simulink model "PARCIAL_2_Sotar_E4"  (R2018a)
settings: Solver=ode15s  StartTime=0.0  StopTime=20  RelTol=1e-3
values from neighbouring files (symbols this model uses):
  L = lqr(A', C', Q, R)'    [PARCIAL_2_E3_script_2p.m]    (also in PARCIAL_2_Sotar_E3.m)
libraries: fl_lib x14, nesl_utility x12, sdolib x5, simulink x5
settings Model: Creator=joses  LastModifiedBy=mluser

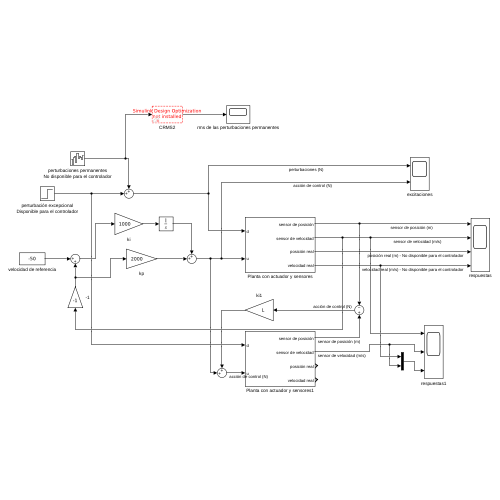
[thumbnail: Simulink's stored preview of the top-level diagram]
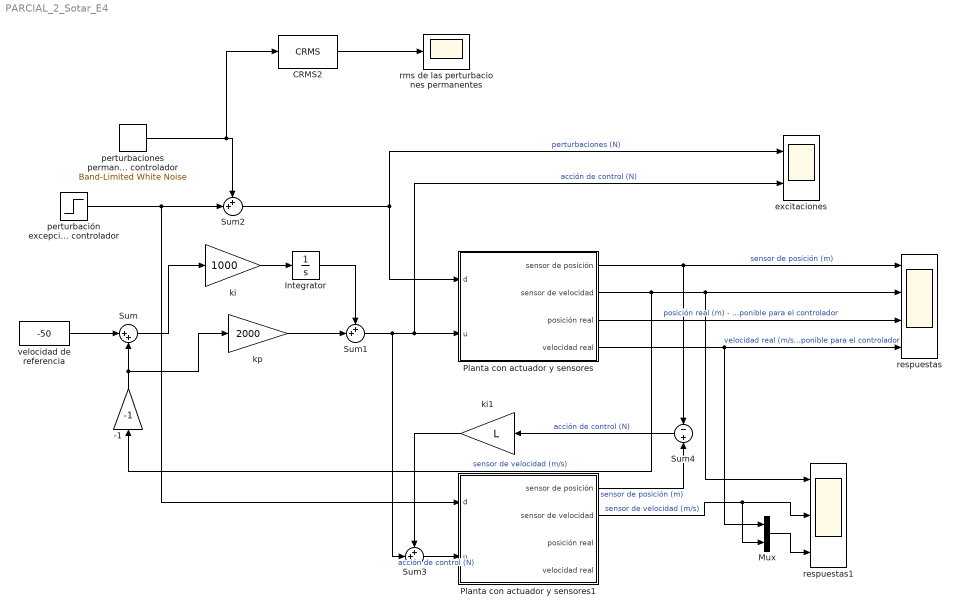
== system PARCIAL_2_Sotar_E4 ==
  -1 : Gain  Gain=-1
  CRMS2 : sdolib/RMS Blocks/CRMS
  Integrator : Integrator
  Mux : Mux  Inputs=2
  Planta con actuador y sensores : Subsystem
  Planta con actuador y sensores1 : Subsystem
  Sum : Sum  Inputs=|++
  Sum1 : Sum  Inputs=++|
  Sum2 : Sum  Inputs=++|
  Sum3 : Sum  Inputs=++|
  Sum4 : Sum  Inputs=-+
  excitaciones : Scope  NumInputPorts=2
  ki : Gain  Gain=1000
  ki1 : Gain  Gain=L
  kp : Gain  Gain=2000
  perturbaciones permanentes No disponible para el controlador : simulink/Sources/Band-Limited White Noise  Cov=100000  Ts=0.01  seed=[23341]
  perturbación excepcional Disponible para el controlador : Step  Time=10  After=20000  SampleTime=0
  respuestas : Scope  NumInputPorts=4
  respuestas1 : Scope  NumInputPorts=3
  rms de las perturbaciones permanentes : Scope
  velocidad de referencia : Constant  Value=-50
  wires:
  Planta con actuador y sensores/2(sensor de velocidad) -> -1/1, respuestas1/1, respuestas/2  "sensor de velocidad (m/s)"
  Planta con actuador y sensores/1(sensor de posición) -> Sum4/1, respuestas/1  "sensor de posición (m)"
  velocidad de referencia/1 -> Sum/1
  Sum/1 -> ki/1
  kp/1 -> Sum1/2
  Planta con actuador y sensores/3(posición real) -> respuestas/3  "posición real (m) - No disponible para el controlador"
  Planta con actuador y sensores/4(velocidad real) -> respuestas/4, Mux/1  "velocidad real (m/s) - No disponible para el controlador"
  Sum1/1 -> Sum3/2, excitaciones/2, Planta con actuador y sensores/2(u)  "acción de control (N)"
  Integrator/1 -> Sum1/1
  ki/1 -> Integrator/1
  perturbación excepcional Disponible para el controlador/1 -> Planta con actuador y sensores1/1(d), Sum2/2
  Sum2/1 -> excitaciones/1, Planta con actuador y sensores/1(d)  "perturbaciones (N)"
  -1/1 -> kp/1, Sum/2
  CRMS2/1 -> rms de las perturbaciones permanentes/1
  perturbaciones permanentes No disponible para el controlador/1 -> CRMS2/1, Sum2/1
  ki1/1 -> Sum3/1
  Planta con actuador y sensores1/1(sensor de posición) -> Sum4/2  "sensor de posición (m)"
  Sum4/1 -> ki1/1  "acción de control (N)"
  Sum3/1 -> Planta con actuador y sensores1/2(u)  "acción de control (N)"
  Planta con actuador y sensores1/2(sensor de velocidad) -> Mux/2, respuestas1/2  "sensor de velocidad (m/s)"
  Mux/1 -> respuestas1/3

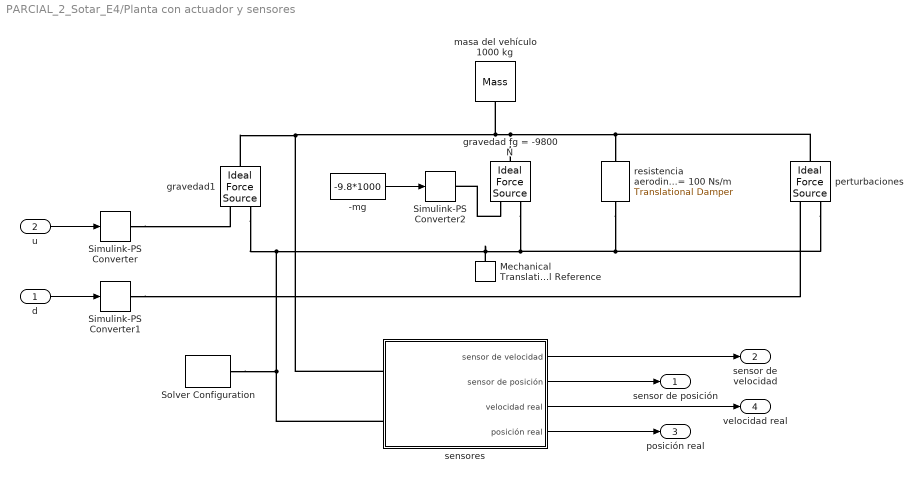
== system PARCIAL_2_Sotar_E4/Planta con actuador y sensores ==
  d : Inport
  u : Inport  Port=2
  -mg : Constant  Value=-9.8*1000
  Mechanical Translational Reference : fl_lib/Mechanical/Translational Elements/Mechanical Translational Reference
  Simulink-PS Converter : nesl_utility/Simulink-PS Converter  PhysicalDomain=network_engine_domain  SubClassName=ps_input  LeftPortType=input  RightPortType=output  PseudoPeriodic=off  Frequencies=[]  NoiseDistribution=none  NoiseParameters=[]  Unit=1  AffineConversion=off  FilteringAndDerivatives=provide  SimscapeFilterOrder=1  InputFilterTimeConstant=0.001  UdotUserProvided=0
  Simulink-PS Converter1 : nesl_utility/Simulink-PS Converter  PhysicalDomain=network_engine_domain  SubClassName=ps_input  LeftPortType=input  RightPortType=output  PseudoPeriodic=off  Frequencies=[]  NoiseDistribution=none  NoiseParameters=[]  Unit=1  AffineConversion=off  FilteringAndDerivatives=provide  SimscapeFilterOrder=1  InputFilterTimeConstant=0.001  UdotUserProvided=0
  Simulink-PS Converter2 : nesl_utility/Simulink-PS Converter  PhysicalDomain=network_engine_domain  SubClassName=ps_input  LeftPortType=input  RightPortType=output  PseudoPeriodic=off  Frequencies=[]  NoiseDistribution=none  NoiseParameters=[]  Unit=1  AffineConversion=off  FilteringAndDerivatives=provide  SimscapeFilterOrder=1  InputFilterTimeConstant=0.001  UdotUserProvided=0
  Solver Configuration : nesl_utility/Solver Configuration  PhysicalDomain=network_engine_domain  SubClassName=solver  LeftPortType=input  RightPortType=generic  Tones=[]  Harmonics=[]  SimulateNoise=off  Profile=off  UseLocalSampling=off  EnableSwitchedLinearOptims=on  FrequencyDomain=off  UseCCode=off  RelTol=0.001  AbsTol=1e-06  MinStep=1e-09  ToWorkspace=off  RevertToSquareIcSolve=off  NumHomotopyIterations=100  PhasorMode=off  PhasorModeNumHarmonics=1  DoDC=off  ResidualTolerance=1e-09  UseLocalSolver=off  LocalSolverChoice=NE_BACKWARD_EULER_ADVANCER  LocalSolverSampleTime=0.001  DoFixedCost=off  MaxNonlinIter=3  MaxModeIter=2  LinearAlgebra=Sparse  EquationFormulation=NE_TIME_EF  DelaysMemoryBudget=1024  AutomaticFiltering=on  FilteringTimeConstant=0.001
  gravedad fg = -9800 N : fl_lib/Mechanical/Mechanical Sources/Ideal Force Source
  gravedad1 : fl_lib/Mechanical/Mechanical Sources/Ideal Force Source
  masa del vehículo 1000 kg : fl_lib/Mechanical/Translational Elements/Mass  mass=1000 kg  v_specify=off  v_priority=High  v=0 m/s  v_nominal_specify=off  v_nominal_unit=m/s  v_nominal_value=1  f_specify=off  f_priority=None  f=0 N  f_nominal_specify=off  f_nominal_unit=N  f_nominal_value=1
  perturbaciones : fl_lib/Mechanical/Mechanical Sources/Ideal Force Source
  resistencia aerodinámica c = 100 Ns/m : fl_lib/Mechanical/Translational Elements/Translational Damper  D=100 N/(m/s)  v_specify=off  v_priority=None  v=0 m/s  v_nominal_specify=off  v_nominal_unit=m/s  v_nominal_value=1  f_specify=off  f_priority=None  f=0 N  f_nominal_specify=off  f_nominal_unit=N  f_nominal_value=1
  sensores : Subsystem
  sensor de posición : Outport  VectorParamsAs1DForOutWhenUnconnected=off
  sensor de velocidad : Outport  Port=2  VectorParamsAs1DForOutWhenUnconnected=off
  posición real : Outport  Port=3  VectorParamsAs1DForOutWhenUnconnected=off
  velocidad real : Outport  Port=4  VectorParamsAs1DForOutWhenUnconnected=off
  wires:
  sensores/2(sensor de posición) -> sensor de posición/1
  sensores/1(sensor de velocidad) -> sensor de velocidad/1
  d/1 -> Simulink-PS Converter1/1
  u/1 -> Simulink-PS Converter/1
  -mg/1 -> Simulink-PS Converter2/1
  sensores/3(velocidad real) -> velocidad real/1
  sensores/4(posición real) -> posición real/1
  connections:
  masa del vehículo 1000 kg/LConn1 -- gravedad1/LConn1 -- sensores/LConn1 -- gravedad fg = -9800 N/LConn1 -- perturbaciones/LConn1 -- resistencia aerodinámica c = 100 Ns/m/RConn1
  Simulink-PS Converter1/RConn1 -- perturbaciones/RConn1
  Mechanical Translational Reference/LConn1 -- gravedad1/RConn2 -- Solver Configuration/RConn1 -- sensores/LConn2 -- resistencia aerodinámica c = 100 Ns/m/LConn1 -- perturbaciones/RConn2 -- gravedad fg = -9800 N/RConn2
  Simulink-PS Converter/RConn1 -- gravedad1/RConn1
  gravedad fg = -9800 N/RConn1 -- Simulink-PS Converter2/RConn1

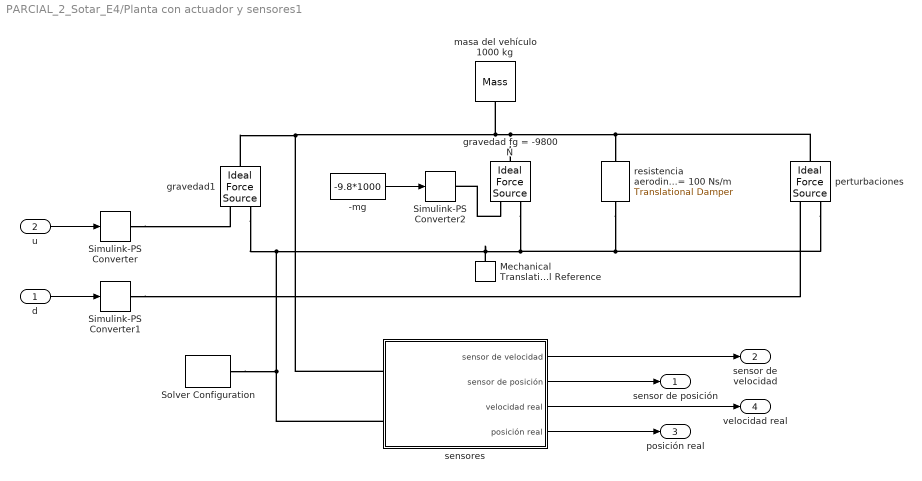
== system PARCIAL_2_Sotar_E4/Planta con actuador y sensores1 ==
  d : Inport
  u : Inport  Port=2
  -mg : Constant  Value=-9.8*1000
  Mechanical Translational Reference : fl_lib/Mechanical/Translational Elements/Mechanical Translational Reference
  Simulink-PS Converter : nesl_utility/Simulink-PS Converter  PhysicalDomain=network_engine_domain  SubClassName=ps_input  LeftPortType=input  RightPortType=output  PseudoPeriodic=off  Frequencies=[]  NoiseDistribution=none  NoiseParameters=[]  Unit=1  AffineConversion=off  FilteringAndDerivatives=provide  SimscapeFilterOrder=1  InputFilterTimeConstant=0.001  UdotUserProvided=0
  Simulink-PS Converter1 : nesl_utility/Simulink-PS Converter  PhysicalDomain=network_engine_domain  SubClassName=ps_input  LeftPortType=input  RightPortType=output  PseudoPeriodic=off  Frequencies=[]  NoiseDistribution=none  NoiseParameters=[]  Unit=1  AffineConversion=off  FilteringAndDerivatives=provide  SimscapeFilterOrder=1  InputFilterTimeConstant=0.001  UdotUserProvided=0
  Simulink-PS Converter2 : nesl_utility/Simulink-PS Converter  PhysicalDomain=network_engine_domain  SubClassName=ps_input  LeftPortType=input  RightPortType=output  PseudoPeriodic=off  Frequencies=[]  NoiseDistribution=none  NoiseParameters=[]  Unit=1  AffineConversion=off  FilteringAndDerivatives=provide  SimscapeFilterOrder=1  InputFilterTimeConstant=0.001  UdotUserProvided=0
  Solver Configuration : nesl_utility/Solver Configuration  PhysicalDomain=network_engine_domain  SubClassName=solver  LeftPortType=input  RightPortType=generic  Tones=[]  Harmonics=[]  SimulateNoise=off  Profile=off  UseLocalSampling=off  EnableSwitchedLinearOptims=on  FrequencyDomain=off  UseCCode=off  RelTol=0.001  AbsTol=1e-06  MinStep=1e-09  ToWorkspace=off  RevertToSquareIcSolve=off  NumHomotopyIterations=100  PhasorMode=off  PhasorModeNumHarmonics=1  DoDC=off  ResidualTolerance=1e-09  UseLocalSolver=off  LocalSolverChoice=NE_BACKWARD_EULER_ADVANCER  LocalSolverSampleTime=0.001  DoFixedCost=off  MaxNonlinIter=3  MaxModeIter=2  LinearAlgebra=Sparse  EquationFormulation=NE_TIME_EF  DelaysMemoryBudget=1024  AutomaticFiltering=on  FilteringTimeConstant=0.001
  gravedad fg = -9800 N : fl_lib/Mechanical/Mechanical Sources/Ideal Force Source
  gravedad1 : fl_lib/Mechanical/Mechanical Sources/Ideal Force Source
  masa del vehículo 1000 kg : fl_lib/Mechanical/Translational Elements/Mass  mass=1000 kg  v_specify=off  v_priority=High  v=0 m/s  v_nominal_specify=off  v_nominal_unit=m/s  v_nominal_value=1  f_specify=off  f_priority=None  f=0 N  f_nominal_specify=off  f_nominal_unit=N  f_nominal_value=1
  perturbaciones : fl_lib/Mechanical/Mechanical Sources/Ideal Force Source
  resistencia aerodinámica c = 100 Ns/m : fl_lib/Mechanical/Translational Elements/Translational Damper  D=100 N/(m/s)  v_specify=off  v_priority=None  v=0 m/s  v_nominal_specify=off  v_nominal_unit=m/s  v_nominal_value=1  f_specify=off  f_priority=None  f=0 N  f_nominal_specify=off  f_nominal_unit=N  f_nominal_value=1
  sensores : Subsystem
  sensor de posición : Outport  VectorParamsAs1DForOutWhenUnconnected=off
  sensor de velocidad : Outport  Port=2  VectorParamsAs1DForOutWhenUnconnected=off
  posición real : Outport  Port=3  VectorParamsAs1DForOutWhenUnconnected=off
  velocidad real : Outport  Port=4  VectorParamsAs1DForOutWhenUnconnected=off
  wires:
  sensores/2(sensor de posición) -> sensor de posición/1
  sensores/1(sensor de velocidad) -> sensor de velocidad/1
  d/1 -> Simulink-PS Converter1/1
  u/1 -> Simulink-PS Converter/1
  -mg/1 -> Simulink-PS Converter2/1
  sensores/3(velocidad real) -> velocidad real/1
  sensores/4(posición real) -> posición real/1
  connections:
  masa del vehículo 1000 kg/LConn1 -- gravedad1/LConn1 -- sensores/LConn1 -- gravedad fg = -9800 N/LConn1 -- perturbaciones/LConn1 -- resistencia aerodinámica c = 100 Ns/m/RConn1
  Simulink-PS Converter1/RConn1 -- perturbaciones/RConn1
  Mechanical Translational Reference/LConn1 -- gravedad1/RConn2 -- Solver Configuration/RConn1 -- sensores/LConn2 -- resistencia aerodinámica c = 100 Ns/m/LConn1 -- perturbaciones/RConn2 -- gravedad fg = -9800 N/RConn2
  Simulink-PS Converter/RConn1 -- gravedad1/RConn1
  gravedad fg = -9800 N/RConn1 -- Simulink-PS Converter2/RConn1

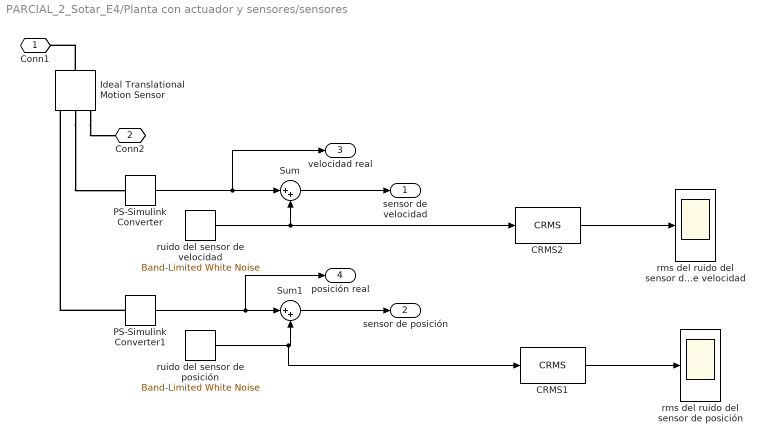
== system PARCIAL_2_Sotar_E4/Planta con actuador y sensores/sensores ==
  CRMS1 : sdolib/RMS Blocks/CRMS
  CRMS2 : sdolib/RMS Blocks/CRMS
  Ideal Translational Motion Sensor : fl_lib/Mechanical/Mechanical Sensors/Ideal Translational Motion Sensor  offset=0 m
  PS-Simulink Converter : nesl_utility/PS-Simulink Converter  PhysicalDomain=network_engine_domain  SubClassName=ps_output  LeftPortType=input  RightPortType=output  PseudoPeriodic=off  Frequencies=[]  Unit=1  AffineConversion=off
  PS-Simulink Converter1 : nesl_utility/PS-Simulink Converter  PhysicalDomain=network_engine_domain  SubClassName=ps_output  LeftPortType=input  RightPortType=output  PseudoPeriodic=off  Frequencies=[]  Unit=1  AffineConversion=off
  Sum : Sum  Inputs=|++
  Sum1 : Sum  Inputs=|++
  rms del ruido del sensor de posición : Scope
  rms del ruido del sensor de velocidad : Scope
  ruido del sensor de posición : simulink/Sources/Band-Limited White Noise  Cov=10  Ts=0.01  seed=[23341]
  ruido del sensor de velocidad : simulink/Sources/Band-Limited White Noise  Cov=1  Ts=0.01  seed=[23341]
  Conn1 : PMIOPort  Side=Left
  Conn2 : PMIOPort  Port=2  Side=Left
  sensor de velocidad : Outport  VectorParamsAs1DForOutWhenUnconnected=off
  sensor de posición : Outport  Port=2  VectorParamsAs1DForOutWhenUnconnected=off
  velocidad real : Outport  Port=3  VectorParamsAs1DForOutWhenUnconnected=off
  posición real : Outport  Port=4  VectorParamsAs1DForOutWhenUnconnected=off
  wires:
  PS-Simulink Converter1/1 -> posición real/1, Sum1/1
  PS-Simulink Converter/1 -> velocidad real/1, Sum/1
  Sum/1 -> sensor de velocidad/1
  Sum1/1 -> sensor de posición/1
  CRMS1/1 -> rms del ruido del sensor de posición/1
  CRMS2/1 -> rms del ruido del sensor de velocidad/1
  ruido del sensor de velocidad/1 -> CRMS2/1, Sum/2
  ruido del sensor de posición/1 -> CRMS1/1, Sum1/2
  connections:
  Ideal Translational Motion Sensor/RConn2 -- PS-Simulink Converter/LConn1
  Ideal Translational Motion Sensor/RConn1 -- Conn2/RConn1
  Ideal Translational Motion Sensor/LConn1 -- Conn1/RConn1
  PS-Simulink Converter1/LConn1 -- Ideal Translational Motion Sensor/RConn3

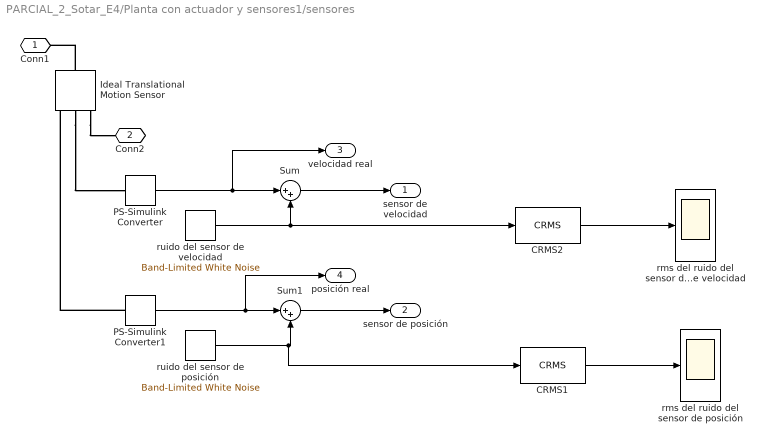
== system PARCIAL_2_Sotar_E4/Planta con actuador y sensores1/sensores ==
  CRMS1 : sdolib/RMS Blocks/CRMS
  CRMS2 : sdolib/RMS Blocks/CRMS
  Ideal Translational Motion Sensor : fl_lib/Mechanical/Mechanical Sensors/Ideal Translational Motion Sensor  offset=0 m
  PS-Simulink Converter : nesl_utility/PS-Simulink Converter  PhysicalDomain=network_engine_domain  SubClassName=ps_output  LeftPortType=input  RightPortType=output  PseudoPeriodic=off  Frequencies=[]  Unit=1  AffineConversion=off
  PS-Simulink Converter1 : nesl_utility/PS-Simulink Converter  PhysicalDomain=network_engine_domain  SubClassName=ps_output  LeftPortType=input  RightPortType=output  PseudoPeriodic=off  Frequencies=[]  Unit=1  AffineConversion=off
  Sum : Sum  Inputs=|++
  Sum1 : Sum  Inputs=|++
  rms del ruido del sensor de posición : Scope
  rms del ruido del sensor de velocidad : Scope
  ruido del sensor de posición : simulink/Sources/Band-Limited White Noise  Cov=10  Ts=0.01  seed=[23341]
  ruido del sensor de velocidad : simulink/Sources/Band-Limited White Noise  Cov=1  Ts=0.01  seed=[23341]
  Conn1 : PMIOPort  Side=Left
  Conn2 : PMIOPort  Port=2  Side=Left
  sensor de velocidad : Outport  VectorParamsAs1DForOutWhenUnconnected=off
  sensor de posición : Outport  Port=2  VectorParamsAs1DForOutWhenUnconnected=off
  velocidad real : Outport  Port=3  VectorParamsAs1DForOutWhenUnconnected=off
  posición real : Outport  Port=4  VectorParamsAs1DForOutWhenUnconnected=off
  wires:
  PS-Simulink Converter1/1 -> posición real/1, Sum1/1
  PS-Simulink Converter/1 -> velocidad real/1, Sum/1
  Sum/1 -> sensor de velocidad/1
  Sum1/1 -> sensor de posición/1
  CRMS1/1 -> rms del ruido del sensor de posición/1
  CRMS2/1 -> rms del ruido del sensor de velocidad/1
  ruido del sensor de velocidad/1 -> CRMS2/1, Sum/2
  ruido del sensor de posición/1 -> CRMS1/1, Sum1/2
  connections:
  Ideal Translational Motion Sensor/RConn2 -- PS-Simulink Converter/LConn1
  Ideal Translational Motion Sensor/RConn1 -- Conn2/RConn1
  Ideal Translational Motion Sensor/LConn1 -- Conn1/RConn1
  PS-Simulink Converter1/LConn1 -- Ideal Translational Motion Sensor/RConn3
